simulink model "Atividade_1"  (R2022a)
settings: Solver=VariableStepAuto  StartTime=0.0  StopTime=25  RelTol=1e-3
settings Model: Creator=luanv  LastModifiedBy=luanv

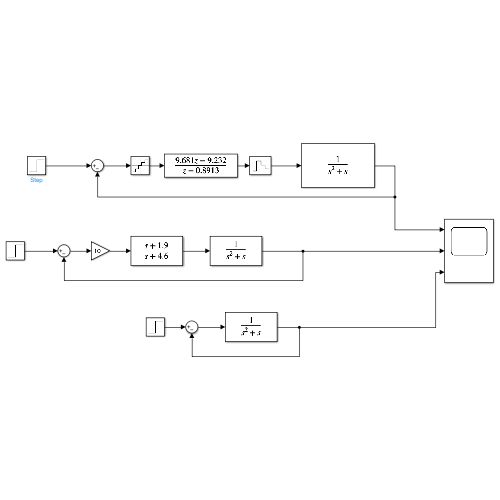
[thumbnail: Simulink's stored preview of the top-level diagram]
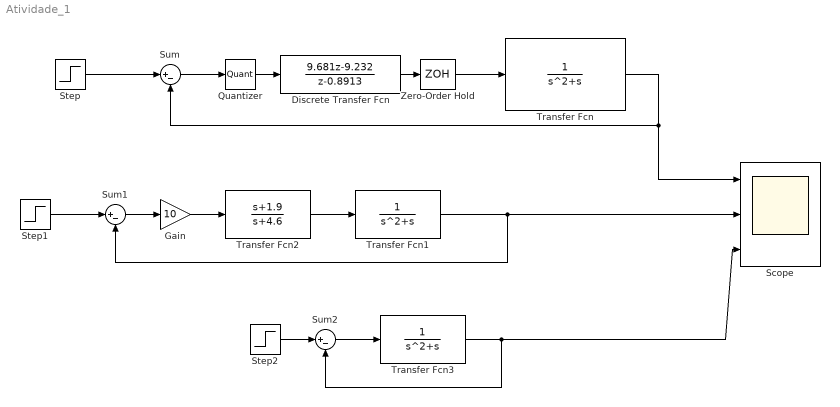
== system Atividade_1 ==
  Discrete Transfer Fcn : DiscreteTransferFcn  Numerator=[9.681 -9.232]  Denominator=[1 -0.8913]
  Gain : Gain  Gain=10
  Quantizer : Quantizer  QuantizationInterval=0.05
  Scope : Scope  NumInputPorts=3
  Step : Step  SampleTime=0
  Step1 : Step  SampleTime=0
  Step2 : Step  SampleTime=0
  Sum : Sum  Inputs=|+-
  Sum1 : Sum  Inputs=|+-
  Sum2 : Sum  Inputs=|+-
  Transfer Fcn : TransferFcn  Denominator=[1 1 0]
  Transfer Fcn1 : TransferFcn  Denominator=[1 1 0]
  Transfer Fcn2 : TransferFcn  Numerator=[1 1.9]  Denominator=[1 4.6]
  Transfer Fcn3 : TransferFcn  Denominator=[1 1 0]
  Zero-Order Hold : ZeroOrderHold  SampleTime=0.025
  wires:
  Sum/1 -> Quantizer/1
  Step/1 -> Sum/1
  Zero-Order Hold/1 -> Transfer Fcn/1
  Transfer Fcn/1 -> Sum/2, Scope/1
  Sum1/1 -> Gain/1
  Step1/1 -> Sum1/1
  Transfer Fcn2/1 -> Transfer Fcn1/1
  Transfer Fcn1/1 -> Sum1/2, Scope/2
  Gain/1 -> Transfer Fcn2/1
  Quantizer/1 -> Discrete Transfer Fcn/1
  Discrete Transfer Fcn/1 -> Zero-Order Hold/1
  Step2/1 -> Sum2/1
  Sum2/1 -> Transfer Fcn3/1
  Transfer Fcn3/1 -> Scope/3, Sum2/2
